simulink model "audiosourceseparation"  (R2021a)
settings: Solver=FixedStepDiscrete  StartTime=0.0  StopTime=Inf  RelTol=1e-3  EnableMultiTasking=on
PreLoadFcn:
  | alpha =linspace(0,1,1e3);
  | sigma = 2 * (alpha - alpha.^2) ./ (alpha.^2 + (1-alpha).^2 );
  | panning = 1 - sigma;
  | panning(1:500) = - panning(1:500);
  | 
  | epsilon = 1e-2;
  | 
  | v = 1e-3;
libraries: dspstat3 x3, dspxfrm3 x2, dspsigops x2, dspindex x2, dspvision x2, dspsnks4 x1, audioutils x1
CloseFcn:
  | clear panning epsilon sigma alpha v
settings Model: Creator=The MathWorks, Inc.  LastModifiedBy=The MathWorks, Inc.
settings SolverCC: AlgebraicLoopSolver=TrustRegion
settings DataIOCC: LimitDataPoints=on  SaveFormat=Array  ReturnWorkspaceOutputs=off
settings OptimizationCC: LifeSpan=inf
settings DebuggingCC: SolverPrmCheckMsg=warning  AllowSymbolicDim=off  SFUnexpectedBacktrackingDiag=warning  SFNoUnconditionalDefaultTransitionDiag=warning  SFExecutionAtInitializationDiag=none  SFMachineParentedDataDiag=warning  ArithmeticOperatorsInVariantConditions=warning
settings HardwareCC: ProdBitPerPointer=32  ProdBitPerSizeT=32  ProdBitPerPtrDiffT=32  ProdLargestAtomicFloat=None  ProdIntDivRoundTo=Undefined  ProdEndianess=Unspecified  ProdWordSize=32  ProdHWDeviceType=32-bit Generic
settings ModelReferenceCC: PropagateSignalLabelsOutOfModel=off
settings SFSimCC: SimUseLocalCustomCode=off  CustomCodeUndefinedFunction=UseInterfaceOnly
settings RTWCC: RTWUseLocalCustomCode=off
settings CodeAppCC: StateflowObjectComments=on
settings GRTTargetCC: TargetLangStandard=C89/C90 (ANSI)
settings ConfigComp: CovMetricSettings=dw  CovSaveCumulativeToWorkspaceVar=on  CovSaveSingleToWorkspaceVar=on  CovExternalEMLEnable=off  CovSFcnEnable=off

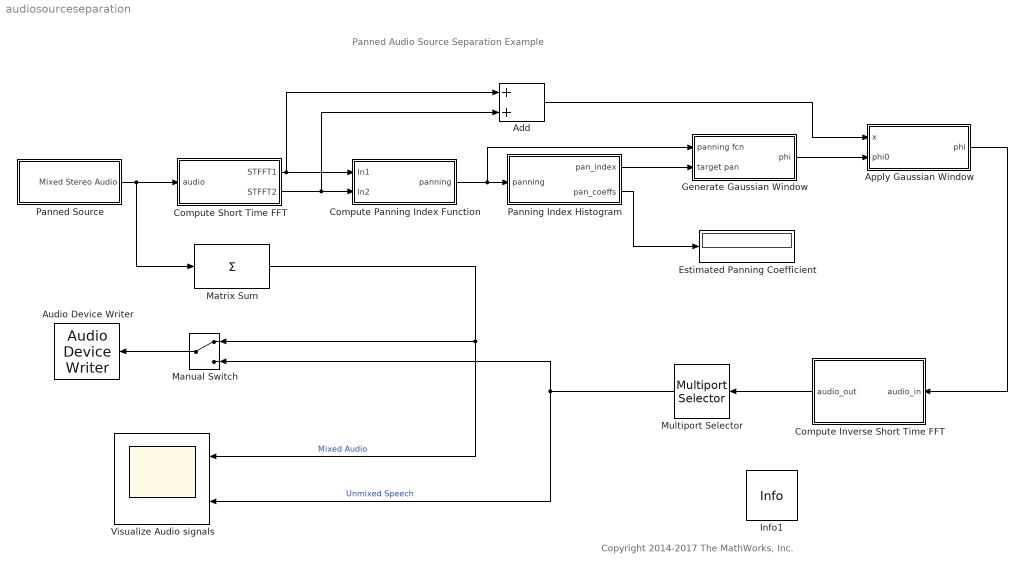
== system audiosourceseparation ==
  note: Panned Audio Source Separation Example
  note: Copyright 2014-2017 The MathWorks, Inc.
  Add : Sum
  Apply Gaussian Window : Subsystem  TreatAsAtomicUnit=on
  Audio Device Writer : dspsnks4/Audio Device Writer  Driver=CoreAudio  Device=Default  InheritSampleRate=on  SampleRate=44100  BitDepth=16-bit integer  BufferSize=4096  NumBuffers=10  DefaultOutputChannelMapping=on  OutputChannelMapping=1:2  OutputNumUnderrunSamples=off  DriverIdx=5  DeviceWarnFlag=''
  Compute Inverse Short Time FFT : Subsystem  TreatAsAtomicUnit=on
  Compute Panning Index Function : Subsystem  TreatAsAtomicUnit=on
  Compute Short Time FFT : Subsystem  TreatAsAtomicUnit=on
  Estimated Panning Coefficient : Display
  Generate Gaussian Window : Subsystem  TreatAsAtomicUnit=on
  Info1 : audioutils/Info  SystemSampleTime=-1  VariantActivationTime=update diagram  Latency=0  AutoFrameSizeCalculation=off
      settings: SourceProductBaseCode=AU
  Manual Switch : ManualSwitch
  Matrix Sum : Sum  Inputs=+  CollapseMode=Specified dimension  CollapseDim=2
  Multiport Selector : dspindex/Multiport Selector  rowsOrCols=Columns  idxCellArray={1}  idxErrMode=Clip Index
  Panned Source : Subsystem  TreatAsAtomicUnit=on  mask{pan=0.400}
      mask prompts: pan "Panning Index"
  Panning Index Histogram : Subsystem  TreatAsAtomicUnit=on
  Visualize Audio signals : Scope  NumInputPorts=2
  wires:
  Panned Source/1(Mixed Stereo Audio) -> Matrix Sum/1, Compute Short Time FFT/1(audio)
  Compute Panning Index Function/1(panning) -> Generate Gaussian Window/1(panning fcn), Panning Index Histogram/1(panning)
  Compute Short Time FFT/1(STFFT1) -> Add/1, Compute Panning Index Function/1(In1)
  Compute Short Time FFT/2(STFFT2) -> Add/2, Compute Panning Index Function/2(In2)
  Panning Index Histogram/1(pan_index) -> Generate Gaussian Window/2(target pan)
  Panning Index Histogram/2(pan_coeffs) -> Estimated Panning Coefficient/1
  Generate Gaussian Window/1(phi) -> Apply Gaussian Window/2(phi0)
  Apply Gaussian Window/1(phi) -> Compute Inverse Short Time FFT/1(audio_in)
  Add/1 -> Apply Gaussian Window/1(x)
  Compute Inverse Short Time FFT/1(audio_out) -> Multiport Selector/1
  Multiport Selector/1 -> Manual Switch/2, Visualize Audio signals/2  "Unmixed Speech"
  Matrix Sum/1 -> Manual Switch/1, Visualize Audio signals/1  "Mixed Audio"
  Manual Switch/1 -> Audio Device Writer/1

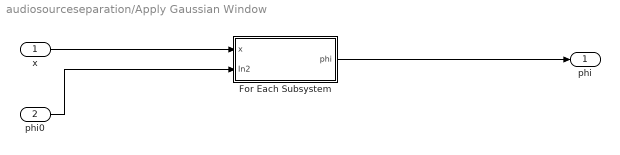
== system audiosourceseparation/Apply Gaussian Window ==
  x : Inport
  phi0 : Inport  Port=2
  For Each Subsystem : Subsystem  TreatAsAtomicUnit=on
  phi : Outport  VectorParamsAs1DForOutWhenUnconnected=off
  wires:
  x/1 -> For Each Subsystem/1(x)
  phi0/1 -> For Each Subsystem/2(In2)
  For Each Subsystem/1(phi) -> phi/1

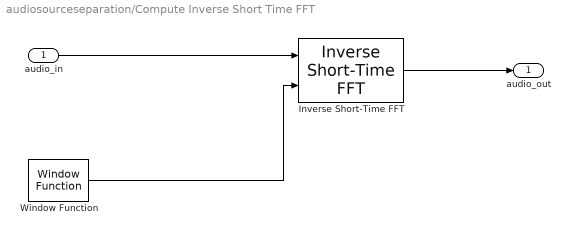
== system audiosourceseparation/Compute Inverse Short Time FFT ==
  audio_in : Inport
  Inverse Short-Time FFT : dspxfrm3/Inverse  Short-Time FFT  W=512  OvLap=384  OutFrameSize=512  InConjSymm=on  DoAssert=off  Tol=1e-4  OutputFrames=off
      settings: SourceProductBaseCode=DS
  Window Function : dspsigops/Window Function  winmode=Generate window  wintype=Hann  sampmode=Discrete  samptime=Inf  N=512  Rs=50  beta=10  winsamp=Symmetric  UserWindow=hamming  OptParams=off  UserParams={'symmetric'}  dataType=double  isSigned=on  wordLen=16  udDataType=sfix(16)  fracBitsMode=Best precision  numFracBits=15  roundingMode=Floor  overflowMode=off  numSidelobes=4  sidelobeLevel=-30
      settings: SourceProductBaseCode=DS
  audio_out : Outport  VectorParamsAs1DForOutWhenUnconnected=off
  wires:
  Window Function/1 -> Inverse Short-Time FFT/2
  audio_in/1 -> Inverse Short-Time FFT/1
  Inverse Short-Time FFT/1 -> audio_out/1

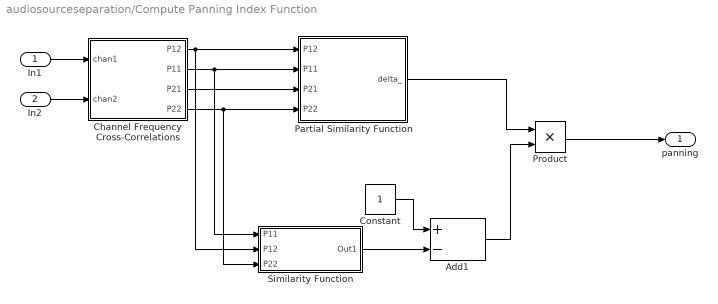
== system audiosourceseparation/Compute Panning Index Function ==
  In1 : Inport
  In2 : Inport  Port=2
  Add1 : Sum  Inputs=+-
  Channel Frequency Cross-Correlations : Subsystem  TreatAsAtomicUnit=on
  Constant : Constant
  Partial Similarity Function : Subsystem  TreatAsAtomicUnit=on
  Product : Product
  Similarity Function : Subsystem
  panning : Outport  VectorParamsAs1DForOutWhenUnconnected=off
  wires:
  Partial Similarity Function/1(delta_) -> Product/1
  Product/1 -> panning/1
  Add1/1 -> Product/2
  Similarity Function/1(Out1) -> Add1/2
  Constant/1 -> Add1/1
  Channel Frequency Cross-Correlations/3(P21) -> Partial Similarity Function/3(P21)
  Channel Frequency Cross-Correlations/2(P11) -> Similarity Function/1(P11), Partial Similarity Function/2(P11)
  Channel Frequency Cross-Correlations/1(P12) -> Similarity Function/2(P12), Partial Similarity Function/1(P12)
  Channel Frequency Cross-Correlations/4(P22) -> Similarity Function/3(P22), Partial Similarity Function/4(P22)
  In1/1 -> Channel Frequency Cross-Correlations/1(chan1)
  In2/1 -> Channel Frequency Cross-Correlations/2(chan2)

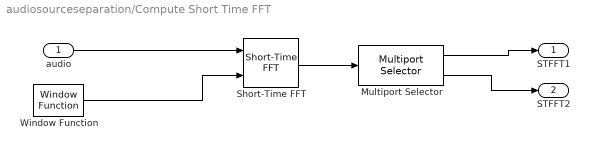
== system audiosourceseparation/Compute Short Time FFT ==
  audio : Inport
  Multiport Selector : dspindex/Multiport Selector  rowsOrCols=Columns  idxCellArray={1,2}  idxErrMode=Clip Index
  Short-Time FFT : dspxfrm3/Short-Time FFT  W=512  OvLap=384  M=1024
      settings: SourceProductBaseCode=DS
  Window Function : dspsigops/Window Function  winmode=Generate window  wintype=Hann  sampmode=Discrete  samptime=Inf  N=512  Rs=50  beta=10  winsamp=Symmetric  UserWindow=hamming  OptParams=off  UserParams={'symmetric'}  dataType=double  isSigned=on  wordLen=16  udDataType=sfix(16)  fracBitsMode=Best precision  numFracBits=15  roundingMode=Floor  overflowMode=off  numSidelobes=4  sidelobeLevel=-30
      settings: SourceProductBaseCode=DS
  STFFT1 : Outport  VectorParamsAs1DForOutWhenUnconnected=off
  STFFT2 : Outport  Port=2  VectorParamsAs1DForOutWhenUnconnected=off
  wires:
  audio/1 -> Short-Time FFT/1
  Window Function/1 -> Short-Time FFT/2
  Short-Time FFT/1 -> Multiport Selector/1
  Multiport Selector/1 -> STFFT1/1
  Multiport Selector/2 -> STFFT2/1

== system audiosourceseparation/Generate Gaussian Window ==
  panning fcn : Inport
  target pan : Inport  Port=2
  For Each Subsystem : Subsystem  TreatAsAtomicUnit=on
  phi : Outport  VectorParamsAs1DForOutWhenUnconnected=off
  wires:
  panning fcn/1 -> For Each Subsystem/1(panning_fcn)
  target pan/1 -> For Each Subsystem/2(target_pan)
  For Each Subsystem/1(phi) -> phi/1

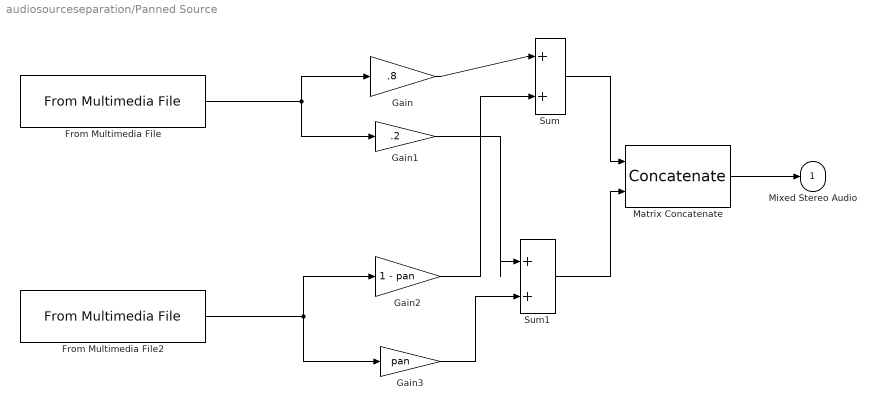
== system audiosourceseparation/Panned Source ==
  From Multimedia File : dspvision/From Multimedia File  inputFilename=TrainWhistle-16-44p1-mono-9secs.wav  readRange=[1 Inf]  loop=on  numPlays=inf  outputStreams=Audio only  videoDataType=single  audioDataType=double  inheritSampleTime=on  userDefinedSampleTime=1/30  noAudioOutput=off  isIntensityVideo=off  fourcc=RGB  colorVideoFormat=Separate color signals  outputEOF=off  dataOrg=Column-major  audioFrameSize=512  computeAudioFrameSize=off  outSamplingMode=Sample based
  From Multimedia File2 : dspvision/From Multimedia File  inputFilename=Counting-16-44p1-mono-15secs.wav  readRange=[1 Inf]  loop=on  numPlays=inf  outputStreams=Audio only  videoDataType=single  audioDataType=double  inheritSampleTime=on  userDefinedSampleTime=1/30  noAudioOutput=off  isIntensityVideo=off  fourcc=RGB  colorVideoFormat=Separate color signals  outputEOF=off  dataOrg=Column-major  audioFrameSize=512  computeAudioFrameSize=off  outSamplingMode=Sample based
  Gain : Gain  Gain=.8
  Gain1 : Gain  Gain=.2
  Gain2 : Gain  Gain=1 - pan
  Gain3 : Gain  Gain=pan
  Matrix Concatenate : Concatenate  Mode=Multidimensional array  ConcatenateDimension=2
  Sum : Sum  Inputs=|++
  Sum1 : Sum  Inputs=|++
  Mixed Stereo Audio : Outport  VectorParamsAs1DForOutWhenUnconnected=off
  wires:
  From Multimedia File/1 -> Gain1/1, Gain/1
  Matrix Concatenate/1 -> Mixed Stereo Audio/1
  Sum/1 -> Matrix Concatenate/1
  Sum1/1 -> Matrix Concatenate/2
  Gain/1 -> Sum/1
  Gain3/1 -> Sum1/2
  From Multimedia File2/1 -> Gain3/1, Gain2/1
  Gain2/1 -> Sum/2
  Gain1/1 -> Sum1/1

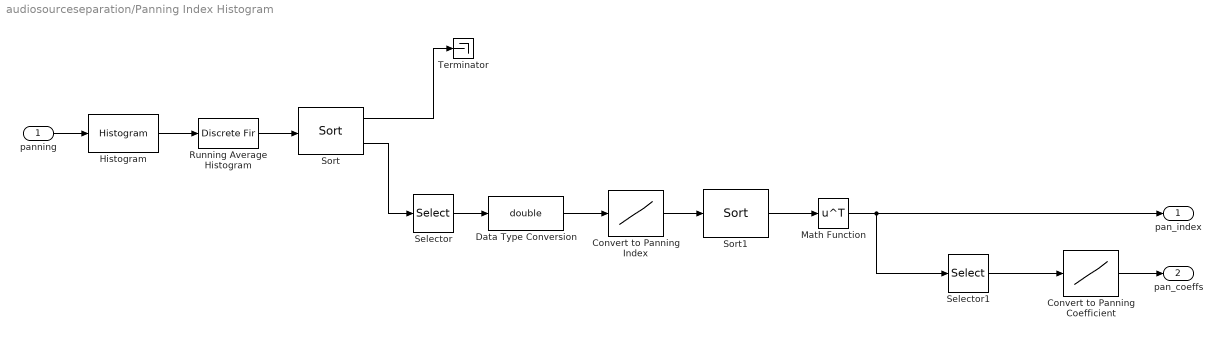
== system audiosourceseparation/Panning Index Histogram ==
  panning : Inport
  Convert to Panning Coefficient : Lookup_n-D  NumberOfTableDimensions=1  BreakpointsForDimension1=panning  Table=linspace(0,1,1e3)  InternalRulePriority=Speed  RndMeth=Simplest  InputSameDT=on
  Convert to Panning Index : Lookup_n-D  NumberOfTableDimensions=1  BreakpointsForDimension1=1:100  Table=linspace(-1,1,1e2)  InternalRulePriority=Speed  RndMeth=Simplest  InputSameDT=on
  Data Type Conversion : DataTypeConversion  OutDataTypeStr=double
  Histogram : dspstat3/Histogram  umin=-1  umax=1  nbins=100  operateOver=Each column  Dimension=1  normalized=on  run=off  reset=on  trigtype=None  colComp=on  roundingMode=Floor  overflowMode=off
      settings: SourceProductBaseCode=DS
  Math Function : Math  Operator=transpose  SignedPower=on  SaturateOnIntegerOverflow=on
  Running Average Histogram : DiscreteFir  Coefficients=ones(1,500)
  Selector : Selector  NumberOfDimensions=2  InputPortWidth=3  IndexOptions=Index vector (dialog),Index vector (dialog)  Indices=[1 2],1  OutputSizes=1,1
  Selector1 : Selector  NumberOfDimensions=2  InputPortWidth=3  IndexOptions=Index vector (dialog),Index vector (dialog)  Indices=1,1  OutputSizes=1,1
  Sort : dspstat3/Sort  otype=Value and Index  dir=Descending  sortAlg=Quick sort  roundingMode=Floor  overflowMode=off  accumDataTypeStr=Inherit: Same as product output  accumLastDataTypeStr=Inherit: Same as product output
      settings: SourceProductBaseCode=DS
  Sort1 : dspstat3/Sort  otype=Value  dir=Descending  sortAlg=Quick sort  roundingMode=Floor  overflowMode=off  accumDataTypeStr=Inherit: Same as product output  accumLastDataTypeStr=Inherit: Same as product output
      settings: SourceProductBaseCode=DS
  Terminator : Terminator
  pan_index : Outport  VectorParamsAs1DForOutWhenUnconnected=off
  pan_coeffs : Outport  Port=2  VectorParamsAs1DForOutWhenUnconnected=off
  wires:
  Sort/2 -> Selector/1
  Sort/1 -> Terminator/1
  panning/1 -> Histogram/1
  Histogram/1 -> Running Average Histogram/1
  Running Average Histogram/1 -> Sort/1
  Convert to Panning Coefficient/1 -> pan_coeffs/1
  Selector/1 -> Data Type Conversion/1
  Convert to Panning Index/1 -> Sort1/1
  Data Type Conversion/1 -> Convert to Panning Index/1
  Sort1/1 -> Math Function/1
  Math Function/1 -> pan_index/1, Selector1/1
  Selector1/1 -> Convert to Panning Coefficient/1

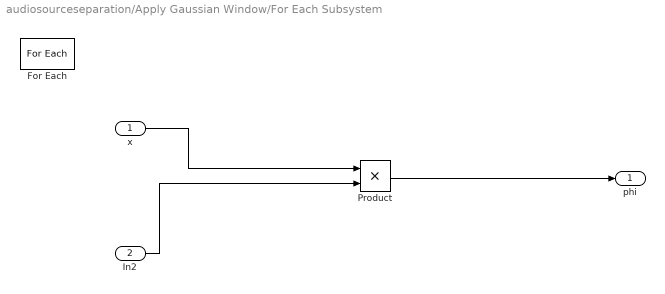
== system audiosourceseparation/Apply Gaussian Window/For Each Subsystem ==
  x : Inport
  In2 : Inport  Port=2  Partition=on  PartitionDimension=2  PartitionWidth=1  PartitionOffset=0
  For Each : ForEach  DisableCoverage=on
  Product : Product
  phi : Outport  ConcatenationDimension=2  VectorParamsAs1DForOutWhenUnconnected=off
  wires:
  x/1 -> Product/1
  In2/1 -> Product/2
  Product/1 -> phi/1

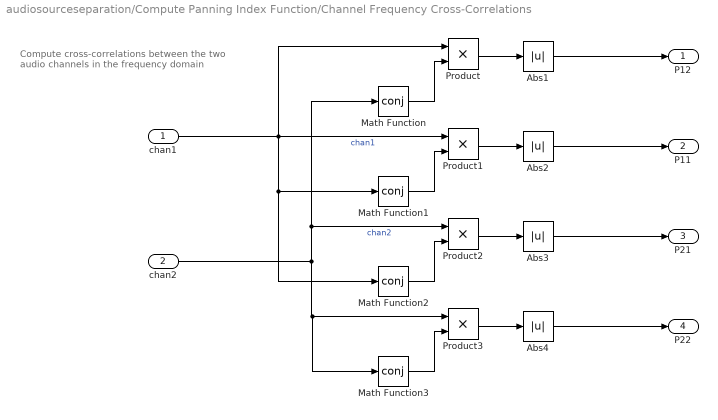
== system audiosourceseparation/Compute Panning Index Function/Channel Frequency Cross-Correlations ==
  note: Compute cross-correlations between
      | the two audio channels in the frequency domain
  chan1 : Inport
  chan2 : Inport  Port=2
  Abs{1..4} (4 alike) : Abs
  Math Function{,1..3} (4 alike) : Math  Operator=conj  SignedPower=on  SaturateOnIntegerOverflow=on
  Product{,1..3} (4 alike) : Product
  P12 : Outport  VectorParamsAs1DForOutWhenUnconnected=off
  P11 : Outport  Port=2  VectorParamsAs1DForOutWhenUnconnected=off
  P21 : Outport  Port=3  VectorParamsAs1DForOutWhenUnconnected=off
  P22 : Outport  Port=4  VectorParamsAs1DForOutWhenUnconnected=off
  wires:
  Math Function/1 -> Product/2
  Product/1 -> Abs1/1
  Math Function1/1 -> Product1/2
  Product1/1 -> Abs2/1
  Math Function2/1 -> Product2/2
  Product2/1 -> Abs3/1
  Math Function3/1 -> Product3/2
  Product3/1 -> Abs4/1
  chan1/1 -> Math Function2/1, Math Function1/1, Product1/1, Product/1  "chan1"
  chan2/1 -> Product2/1, Math Function/1, Math Function3/1, Product3/1  "chan2"
  Abs1/1 -> P12/1
  Abs2/1 -> P11/1
  Abs3/1 -> P21/1
  Abs4/1 -> P22/1

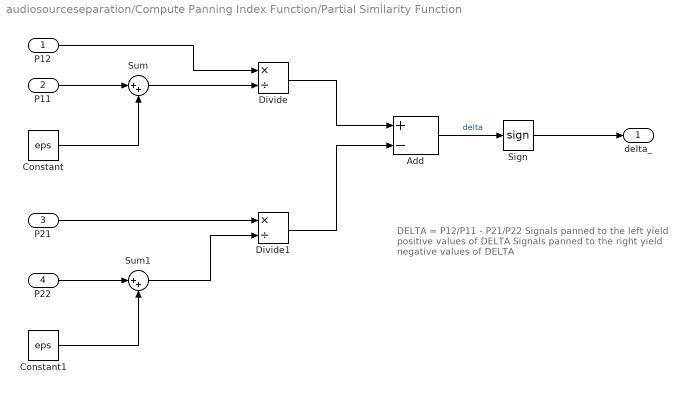
== system audiosourceseparation/Compute Panning Index Function/Partial Similarity Function ==
  note: DELTA = P12/P11 - P21/P22
      |
      | Signals panned to the left yield positive values of DELTA
      |
      | Signals panned to the right yield negative values of DELTA
  P12 : Inport
  P11 : Inport  Port=2
  P21 : Inport  Port=3
  P22 : Inport  Port=4
  Add : Sum  Inputs=+-
  Constant : Constant  Value=eps
  Constant1 : Constant  Value=eps
  Divide : Product  Inputs=*/
  Divide1 : Product  Inputs=*/
  Sign : Signum
  Sum : Sum  Inputs=|++
  Sum1 : Sum  Inputs=|++
  delta_ : Outport  VectorParamsAs1DForOutWhenUnconnected=off
  wires:
  P12/1 -> Divide/1
  P21/1 -> Divide1/1
  P11/1 -> Sum/1
  Sum/1 -> Divide/2
  Constant/1 -> Sum/2
  P22/1 -> Sum1/1
  Sum1/1 -> Divide1/2
  Constant1/1 -> Sum1/2
  Divide/1 -> Add/1
  Divide1/1 -> Add/2
  Add/1 -> Sign/1  "delta"
  Sign/1 -> delta_/1

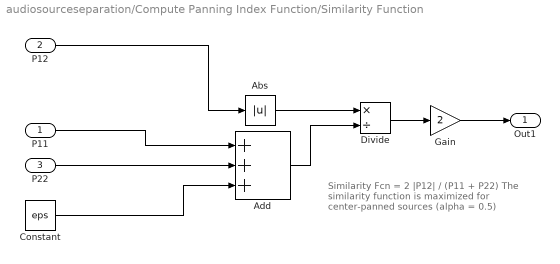
== system audiosourceseparation/Compute Panning Index Function/Similarity Function ==
  note: Similarity Fcn = 2 |P12| / (P11 + P22)
      |
      | The similarity function is maximized for
      | center-panned sources (alpha = 0.5)
  P11 : Inport
  P12 : Inport  Port=2
  P22 : Inport  Port=3
  Abs : Abs
  Add : Sum  Inputs=+++
  Constant : Constant  Value=eps
  Divide : Product  Inputs=*/
  Gain : Gain  Gain=2
  Out1 : Outport  VectorParamsAs1DForOutWhenUnconnected=off
  wires:
  Gain/1 -> Out1/1
  Divide/1 -> Gain/1
  P12/1 -> Abs/1
  Add/1 -> Divide/2
  P22/1 -> Add/2
  P11/1 -> Add/1
  Constant/1 -> Add/3
  Abs/1 -> Divide/1

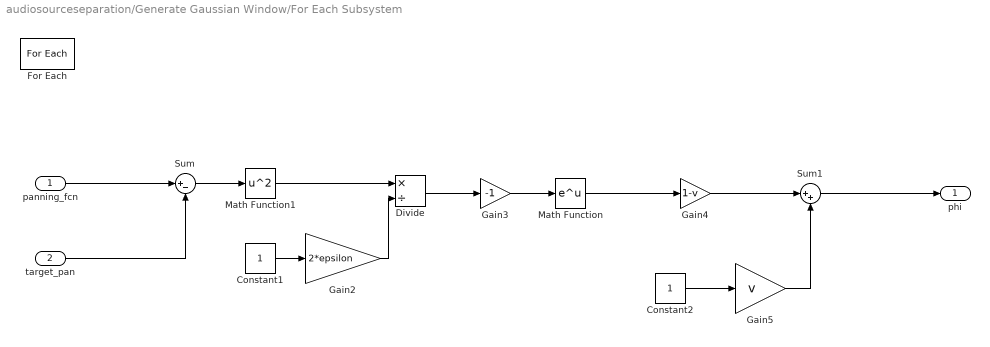
== system audiosourceseparation/Generate Gaussian Window/For Each Subsystem ==
  panning_fcn : Inport
  target_pan : Inport  Port=2  Partition=on  PartitionDimension=2  PartitionWidth=1  PartitionOffset=0
  Constant1 : Constant
  Constant2 : Constant
  Divide : Product  Inputs=*/
  For Each : ForEach  DisableCoverage=on
  Gain2 : Gain  Gain=2*epsilon
  Gain3 : Gain  Gain=-1
  Gain4 : Gain  Gain=1-v
  Gain5 : Gain  Gain=v
  Math Function : Math  SignedPower=on  SaturateOnIntegerOverflow=on
  Math Function1 : Math  Operator=square  SignedPower=on  SaturateOnIntegerOverflow=on
  Sum : Sum  Inputs=|+-
  Sum1 : Sum  Inputs=|++
  phi : Outport  ConcatenationDimension=2  VectorParamsAs1DForOutWhenUnconnected=off
  wires:
  panning_fcn/1 -> Sum/1
  Sum/1 -> Math Function1/1
  Math Function1/1 -> Divide/1
  Constant1/1 -> Gain2/1
  Gain2/1 -> Divide/2
  Divide/1 -> Gain3/1
  Gain3/1 -> Math Function/1
  Math Function/1 -> Gain4/1
  Gain4/1 -> Sum1/1
  Constant2/1 -> Gain5/1
  Gain5/1 -> Sum1/2
  Sum1/1 -> phi/1
  target_pan/1 -> Sum/2
